simulink model "downCounter"  (R2021a)
settings: Solver=ode45  StartTime=0.0  StopTime=10.0  RelTol=1e-3
settings Model: Creator=DELL  LastModifiedBy=DELL

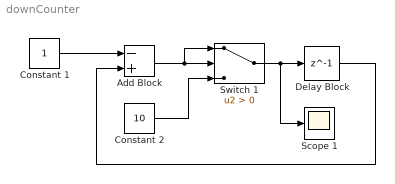
== system downCounter ==
  Add Block : Sum  Inputs=-+
  Constant 1 : Constant  VectorParams1D=off
  Constant 2 : Constant  Value=10  VectorParams1D=off
  Delay Block : Delay  DelayLength=1  InitialCondition=0
  Scope 1 : Scope
  Switch 1 : Switch  Criteria=u2 > Threshold
  wires:
  Delay Block/1 -> Add Block/2
  Constant 2/1 -> Switch 1/3
  Constant 1/1 -> Add Block/1
  Switch 1/1 -> Scope 1/1, Delay Block/1
  Add Block/1 -> Switch 1/2, Switch 1/1
